simulink model "controladorbasico"  (Simulink 7.9)
settings: Solver=ode45  StartTime=0.0  StopTime=100  RelTol=1e-3
settings Model: Creator=Miguel Faggioni  LastModifiedBy=Miguel Faggioni
settings DataIOCC: TimeSaveName=t

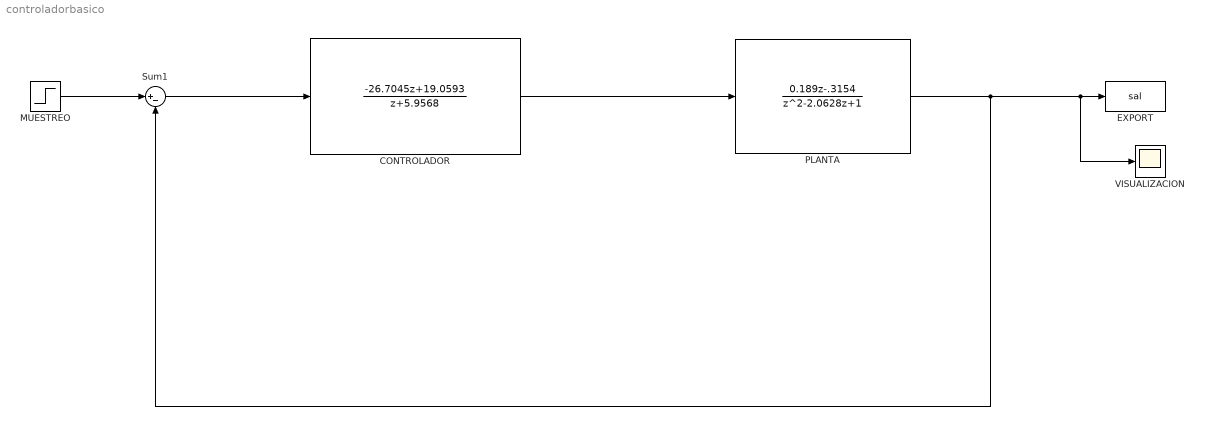
== system controladorbasico ==
  CONTROLADOR : DiscreteTransferFcn  Numerator=[-26.7045 19.0593]  Denominator=[1 5.9568]
  EXPORT : ToWorkspace  VariableName=sal  SampleTime=-1
  MUESTREO : Step  Time=0  After=2  SampleTime=.1
  PLANTA : DiscreteTransferFcn  Numerator=[0.189 -.3154]  Denominator=[1 -2.0628 1]
  Sum1 : Sum  Inputs=|+-
  VISUALIZACION : Scope
      settings: TimeRange=100  YMin=1.73389  YMax=1.91641
  wires:
  MUESTREO/1 -> Sum1/1
  Sum1/1 -> CONTROLADOR/1
  PLANTA/1 -> Sum1/2, EXPORT/1, VISUALIZACION/1
  CONTROLADOR/1 -> PLANTA/1
